simulink model "Project_Sim_Adapt"  (R2025a)
settings: Solver=VariableStepAuto  StartTime=0.0  StopTime=simulation_time  RelTol=1e-3
undefined symbols (not defined in the file): N, omegaB0, pWB0, qWB0, Ts, vWB0, x0, Xref
libraries: robotcorelib x1, uavutilslib x1
settings Model: Creator=franc  LastModifiedBy=franc
settings DebuggingCC: UnderspecifiedInitializationDetection=Classic  MergeDetectMultiDrivingBlocksExec=none
settings ModelReferenceCC: PropagateSignalLabelsOutOfModel=off
settings RTWCC: GPUComputeCapability=3.5

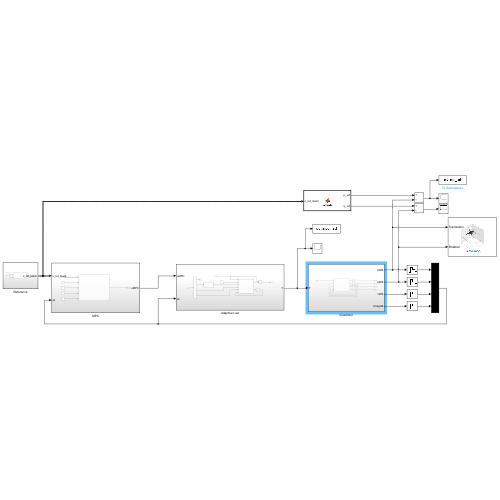
[thumbnail: Simulink's stored preview of the top-level diagram]
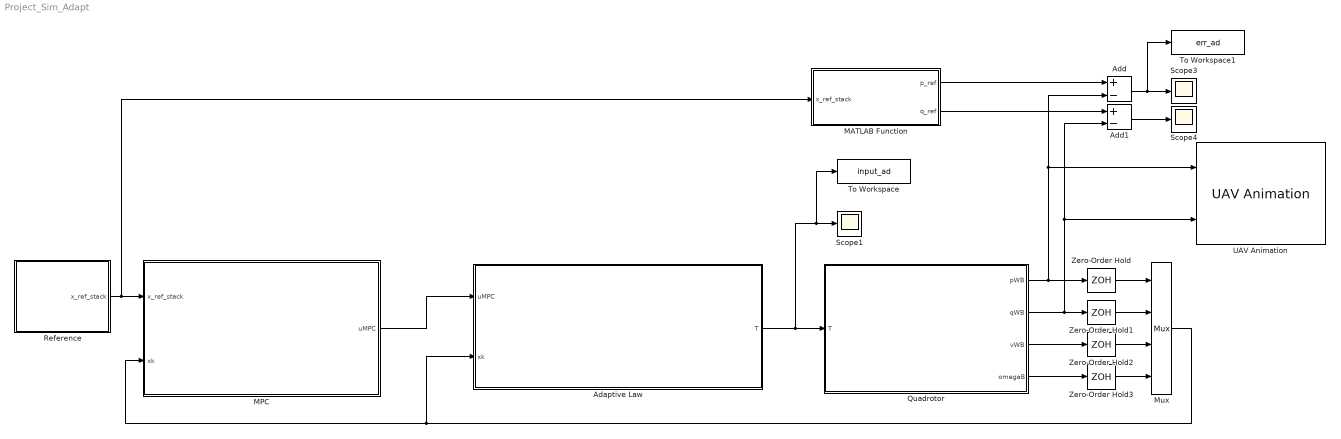
== system Project_Sim_Adapt ==
  Adaptive Law : Subsystem
  Add : Sum  Inputs=+-
  Add1 : Sum  Inputs=+-
  MATLAB Function : MATLAB Function  TreatAsAtomicUnit=on
  MPC : Subsystem
  Mux : Mux
  Quadrotor : Subsystem
  Reference : Subsystem
  Scope1 : Scope
      settings: ActiveDisplayYMinimum=1.7052326467122152  ActiveDisplayYMaximum=1.8134132267959873
  Scope3 : Scope
      settings: ActiveDisplayYMinimum=-0.065328340754687408  ActiveDisplayYMaximum=0.039807612944060038  DataLoggingVariableName=ScopeData4
  Scope4 : Scope
      settings: ActiveDisplayYMinimum=-0.128474772332549  ActiveDisplayYMaximum=0.10839492409722418  DataLoggingVariableName=ScopeData5
  To Workspace : ToWorkspace  VariableName=input_ad  SaveFormat=Structure With Time  SampleTime=-1
  To Workspace1 : ToWorkspace  VariableName=err_ad  SaveFormat=Structure With Time  SampleTime=-1
  UAV Animation : uavutilslib/UAV Animation  NumUAV=1  DynamicUAVConfig=off  UAVType=Multirotor  UAVSize=1  UAVColor=[1 0 0]  UAVTrajectoryAlpha=1  InertialZDirection=Up  RotationFormat=Quaternion  DrawMarkers=off  SampleTime=-1
  Zero-Order Hold{,1..3} (4 alike) : ZeroOrderHold  SampleTime=Ts
  wires:
  Quadrotor/1(pWB) -> UAV Animation/1, Add/2, Zero-Order Hold/1
  Quadrotor/2(qWB) -> UAV Animation/2, Add1/2, Zero-Order Hold1/1
  Quadrotor/3(vWB) -> Zero-Order Hold2/1
  Quadrotor/4(omegaB) -> Zero-Order Hold3/1
  Zero-Order Hold3/1 -> Mux/4
  Zero-Order Hold2/1 -> Mux/3
  Zero-Order Hold1/1 -> Mux/2
  Zero-Order Hold/1 -> Mux/1
  Mux/1 -> Adaptive Law/2(xk), MPC/2(xk)
  Reference/1(x_ref_stack) -> MATLAB Function/1(x_ref_stack), MPC/1(x_ref_stack)
  MATLAB Function/1(p_ref) -> Add/1
  Add/1 -> To Workspace1/1, Scope3/1
  MATLAB Function/2(q_ref) -> Add1/1
  Add1/1 -> Scope4/1
  Adaptive Law/1(T) -> To Workspace/1, Scope1/1, Quadrotor/1(T)
  MPC/1(uMPC) -> Adaptive Law/1(uMPC)

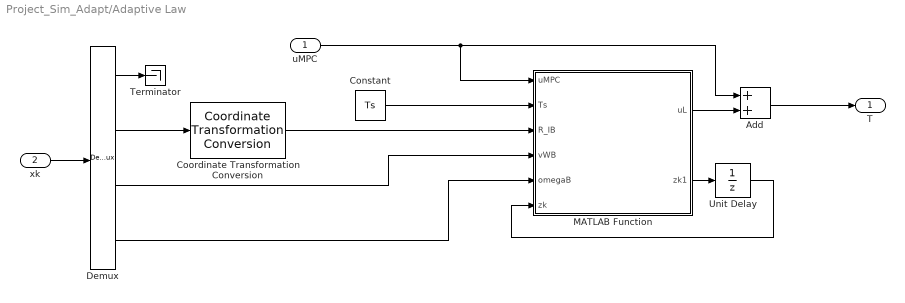
== system Project_Sim_Adapt/Adaptive Law ==
  uMPC : Inport
  xk : Inport  Port=2
  Add : Sum
  Constant : Constant  Value=Ts
  Coordinate Transformation Conversion : robotcorelib/Coordinate Transformation Conversion  InputRepresentation=Quaternion  InputEulerSequence=ZYX  ShowTrVecInputPort=on  OutputRepresentation=Rotation Matrix  OutputEulerSequence=ZYX  ShowTrVecOutputPort=on  SimulateUsing=Interpreted execution
      settings: LibrarySourceBlock=uavutilslib/Coordinate Transformation Conversion
  Demux : Demux  Outputs=[3 4 3 3]
  MATLAB Function : MATLAB Function  TreatAsAtomicUnit=on
  Terminator : Terminator
  Unit Delay : UnitDelay  SampleTime=-1  HasFrameUpgradeWarning=on
  T : Outport
  wires:
  xk/1 -> Demux/1
  Demux/3 -> MATLAB Function/4(vWB)
  Demux/4 -> MATLAB Function/5(omegaB)
  uMPC/1 -> Add/1, MATLAB Function/1(uMPC)
  Demux/1 -> Terminator/1
  Constant/1 -> MATLAB Function/2(Ts)
  Coordinate Transformation Conversion/1 -> MATLAB Function/3(R_IB)
  MATLAB Function/2(zk1) -> Unit Delay/1
  Unit Delay/1 -> MATLAB Function/6(zk)
  Demux/2 -> Coordinate Transformation Conversion/1
  MATLAB Function/1(uL) -> Add/2
  Add/1 -> T/1

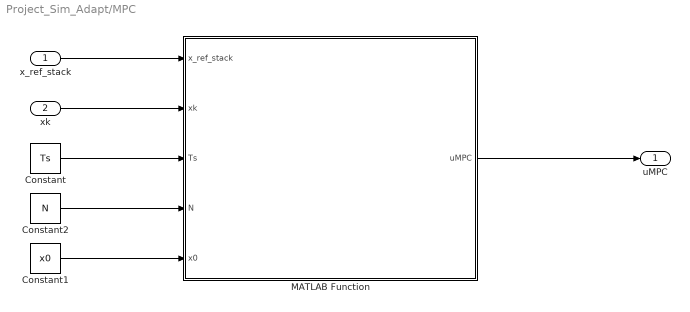
== system Project_Sim_Adapt/MPC ==
  x_ref_stack : Inport
  xk : Inport  Port=2
  Constant : Constant  Value=Ts
  Constant1 : Constant  Value=x0
  Constant2 : Constant  Value=N
  MATLAB Function : MATLAB Function  TreatAsAtomicUnit=on
  uMPC : Outport
  wires:
  Constant/1 -> MATLAB Function/3(Ts)
  Constant1/1 -> MATLAB Function/5(x0)
  xk/1 -> MATLAB Function/2(xk)
  MATLAB Function/1(uMPC) -> uMPC/1
  Constant2/1 -> MATLAB Function/4(N)
  x_ref_stack/1 -> MATLAB Function/1(x_ref_stack)

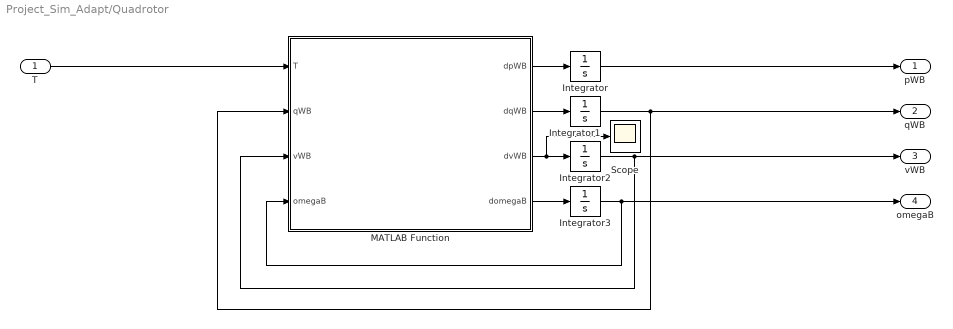
== system Project_Sim_Adapt/Quadrotor ==
  T : Inport
  Integrator : Integrator  InitialCondition=pWB0
  Integrator1 : Integrator  InitialCondition=qWB0
  Integrator2 : Integrator  InitialCondition=vWB0
  Integrator3 : Integrator  InitialCondition=omegaB0
  MATLAB Function : MATLAB Function  TreatAsAtomicUnit=on
  Scope : Scope
      settings: ActiveDisplayYMinimum=-10.516652542372883  ActiveDisplayYMaximum=1.7458474576271188  DataLoggingVariableName=ScopeData2
  pWB : Outport
  qWB : Outport  Port=2
  vWB : Outport  Port=3
  omegaB : Outport  Port=4
  wires:
  T/1 -> MATLAB Function/1(T)
  MATLAB Function/1(dpWB) -> Integrator/1
  MATLAB Function/2(dqWB) -> Integrator1/1
  MATLAB Function/3(dvWB) -> Scope/1, Integrator2/1
  MATLAB Function/4(domegaB) -> Integrator3/1
  Integrator1/1 -> MATLAB Function/2(qWB), qWB/1
  Integrator2/1 -> MATLAB Function/3(vWB), vWB/1
  Integrator3/1 -> MATLAB Function/4(omegaB), omegaB/1
  Integrator/1 -> pWB/1

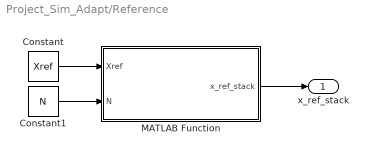
== system Project_Sim_Adapt/Reference ==
  Constant : Constant  Value=Xref
  Constant1 : Constant  Value=N
  MATLAB Function : MATLAB Function  TreatAsAtomicUnit=on  SystemSampleTime=Ts
  x_ref_stack : Outport
  wires:
  Constant1/1 -> MATLAB Function/2(N)
  Constant/1 -> MATLAB Function/1(Xref)
  MATLAB Function/1(x_ref_stack) -> x_ref_stack/1

== matlab function Project_Sim_Adapt/MPC/MATLAB Function ==
  data: x_ref_stack input; xk input size=13; uMPC output size=4; Ts input size=1; N input; x0 input size=13
function uMPC = MPC(x_ref_stack,xk,Ts,N,x0)

% Initialization
persistent ubar x0_guess u0_guess;

u_hover = 0.716*9.81/4; 
if isempty(ubar)
    ubar = u_hover*ones(4,1);
end

% Dimensions
nx = 13;
nu = 4;

% Cost parameters
R = 10*eye(nu);
Q = diag(400*[10 10 200 1 1 1 1 1 1 1 1 1 1]);

% Inequality constraints per time step (input) (H_u*u <= k_u)
rpm_max = 10880;
omega_max = rpm_max*2*pi/60;
u_max = 1.6e-2*omega_max^2;

H_u = [ eye(nu);
      -eye(nu)];
k_u = [ u_max*ones(nu,1);
       zeros(nu,1)];

% Inequality constraints per time step (state, fictional) (H_x*x <= k_x)
x_min = -1e6*ones(nx,1);
x_max = 1e6*ones(nx,1);
H_x = [ eye(nx);
       -eye(nx)];
k_x = [ x_max;
       -x_min ];

% System dynamics (Computation of the linearized system around the current state)
[Ak,Bk,ck] = lin_fdyn_central(xk, ubar, Ts);

% Inequality constraints for the whole horizon (A*z <= b)
% z = [x0,x1,...,xN-1,xN,u0,u1,...,uN-1]'
Ax = kron(eye(N+1), H_x);
bx = repmat(k_x, N+1, 1);
Au = kron(eye(N), H_u);
bu = repmat(k_u, N, 1);

A = blkdiag(Ax,Au);
b = [bx;bu];

% Equality constraints
Aeq=zeros(nx*(N+1),nx*(N+1)+nu*N);
beq=zeros(nx*(N+1),1);

for k=0:N-1 % Linearized system dynamics constraints 
    Aeq(nx*k+1:nx*(k+1),1:nx*(N+1))=[zeros(nx,nx*k),Ak,-eye(nx),zeros(nx,nx*(N-1-k))];
    Aeq(nx*k+1:nx*(k+1),nx*(N+1)+1:end)=[zeros(nx,nu*k),Bk,zeros(nx,nu*(N-1-k))];
    beq(nx*k+1:nx*(k+1)) = -ck;
end

% Initial condition constraints
Aeq(nx*N+1:nx*(N+1),:)=[eye(nx),zeros(nx,nu*N+nx*N)];
beq(nx*N+1:nx*(N+1))=xk;

% Cost function
Qstack = kron(eye(N+1), Q); % Q, but for the whole horizon
Rstack = kron(eye(N), R); % R, but for the whole horizon
    
HQP = blkdiag(Qstack,Rstack); % Overall cost

u_ref_stack = repmat(u_hover*ones(nu,1), N, 1); % Constant reference on the input
fQP = -HQP * [x_ref_stack; u_ref_stack]; % x and u centered on their references

% solver parameters
if isempty(x0_guess)
    x0_guess = repmat(x0,N+1,1);
end
if isempty(u0_guess)
    u0_guess = repmat(u_hover*ones(nu,1),N,1);
end
tol_opt       = 1e-8;
options = optimoptions('quadprog', ...
                       'Algorithm', 'active-set', ...
                       'MaxIterations', 10000, ...
                       'OptimalityTolerance', tol_opt, ...
                       'StepTolerance', tol_opt);

% optimization
solutionOL = quadprog(HQP,fQP,A,b,Aeq,beq,[],[],[x0_guess;u0_guess],options);

% Derive the optimal predicted state and input sequence
x_OL_tilde = solutionOL(1:nx*(N+1),1);
u_OL_tilde = solutionOL(nx*(N+1)+1:end,1);
x_OL = reshape(x_OL_tilde,nx,N+1);
u_OL = reshape(u_OL_tilde,nu,N);

% Prepare warmstart solution for next time step 
x0_guess = [x_OL_tilde(nx+1:end);zeros(nx,1)];
u0_guess = [u_OL_tilde(nu+1:end);zeros(nu,1)];

% Imposing MPC action
uMPC = u_OL(:,1);
ubar = uMPC;

%% functions for system dynamics

    function [Ak,Bk,ck] = lin_fdyn_central(xbar, ubar, dt) % system dynamics linearization

        % Retrieving the Nonlinear system dynamics
        nnx = numel(xbar);
        nnu = numel(ubar);
        f0 = fRK4(xbar, ubar, dt);

        % denominator settings
        hx = (eps^(1/3))*max(1, abs(xbar));
        hu = (eps^(1/3))*max(1, abs(ubar));

        % Matrices initialization
        Ak = zeros(nnx);
        Bk = zeros(nnx,nnu);

        for i = 1:nnx % Ak computation
            dx = zeros(nnx,1);
            dx(i) = hx(i);
            fp = fRK4(xbar+dx, ubar, dt);
            fm = fRK4(xbar-dx, ubar, dt);
            Ak(:,i) = (fp-fm)/(2*hx(i));
        end

        for j = 1:nnu % Bk computation
            du = zeros(nnu,1);
            du(j) = hu(j);
            fp = fRK4(xbar, ubar+du, dt);
            fm = fRK4(xbar, ubar-du, dt);
            Bk(:,j) = (fp-fm)/(2*hu(j));
       end

       ck = f0-Ak*xbar-Bk*ubar; % Residual computation
    end


    function xk1 = fRK4(xk,uk,deltaT) % Runge-Kutta 4th order discretization
        k1 = f(xk,uk);
        k2 = f(xk+deltaT/2*k1,uk);
        k3 = f(xk+deltaT/2*k2,uk);
        k4 = f(xk+deltaT*k3,uk);
        xk1 = xk+deltaT/6*(k1+2*k2+2*k3+k4);
    end

    function dotx = f(x,u) % Nonlinear Nominal system dynamics (see Plant code for details)
    g = 9.81;
    g_vec = [0 0 -g]';

    T0 = u(1);
    T1 = u(2);
    T2 = u(3);
    T3 = u(4);

    TB = [0 0 T0+T1+T2+T3]';
    m = 0.716;
    
    Jx = 0.007;
    Jy = Jx;
    Jz = 0.012;

    J = diag([Jx,Jy,Jz]);

    xx = zeros(4,1);
    yy = zeros(4,1);
    dxx = zeros(4,1);
    dyy = zeros(4,1);

    l = 0.17;
    theta = [0 pi/2 pi -pi/2]';
    for i=1:4
       xx(i)=l*cos(theta(i));
       yy(i)=l*sin(theta(i));
    end
    for i=1:4
        dxx(i)=abs(yy(i));
        dyy(i)=abs(xx(i));
    end
    cT = 1.6e-2;
    P = [-dxx(1) -dxx(2) dxx(3) dxx(4);
         dyy(1) -dyy(2) -dyy(3) dyy(4)
         -cT     cT    -cT    cT];

    tauB = P*[T0 T1 T2 T3]';

    pWB = x(1:3);
    qWB = x(4:7);
    vWB = x(8:10);
    omegaB = x(11:13);

    dpWB = vWB;
    dqWB = quatmultiply(qWB,[0 omegaB'/2]');
    dvWB = quaternion_product(qWB,TB/m)+g_vec;
    domegaB = inv(J)*(tauB - cross(omegaB, J*omegaB));

    dotx = [dpWB;dqWB;dvWB;domegaB];


        function res = quaternion_product(q, vec) % quaternion * vector
        q = q/ norm(q);
        q_conj = [q(1) -q(2) -q(3) -q(4)]';
        q_vec = [0 vec']';
        res = quatmultiply(q, q_vec);
        res = quatmultiply(res,q_conj);
        res = res(2:4);
    end


    function q_out = quatmultiply(q1, q2) % quaternion multiplication

    qw1 = q1(1); qx1 = q1(2); qy1 = q1(3); qz1 = q1(4);
    qw2 = q2(1); qx2 = q2(2); qy2 = q2(3); qz2 = q2(4);

    q_out = [qw1*qw2 - qx1*qx2 - qy1*qy2 - qz1*qz2; 
             qw1*qx2 + qx1*qw2 + qy1*qz2 - qz1*qy2; 
             qw1*qy2 - qx1*qz2 + qy1*qw2 + qz1*qx2; 
             qw1*qz2 + qx1*qy2 - qy1*qx2 + qz1*qw2];
    end
    end
end

== matlab function Project_Sim_Adapt/Quadrotor/MATLAB Function ==
  data: T input size=4; qWB input size=4; vWB input size=3; dpWB output size=3; dqWB output size=4; dvWB output size=3; domegaB output size=3; omegaB input size=3
function [dpWB,dqWB,dvWB,domegaB] = dynamics(T,qWB,vWB,omegaB)

    % gravity term
    g = 9.81;
    g_vec = [0 0 -g]';

    % thrusts
    T0 = T(1);
    T1 = T(2);
    T2 = T(3);
    T3 = T(4);
    TB = [0 0 T0+T1+T2+T3]';
    
    % mass
    m = 0.716;
    
    % Inertia
    Jx = 0.007;
    Jy = Jx;
    Jz = 0.012;
    J = diag([Jx,Jy,Jz]);

    % Allocation Matrix computation
    l = 0.17;
    theta = [0 pi/2 pi -pi/2]';
    xx = zeros(4,1);
    yy = zeros(4,1);
    dxx = zeros(4,1);
    dyy = zeros(4,1);
    for i=1:4
       xx(i)=l*cos(theta(i));
       yy(i)=l*sin(theta(i));
    end
    for i=1:4
        dxx(i)=abs(yy(i));
        dyy(i)=abs(xx(i));
    end
    cT = 1.6e-2;
    P = [-dxx(1) -dxx(2) dxx(3) dxx(4);
         dyy(1) -dyy(2) -dyy(3) dyy(4)
         -cT     cT    -cT    cT];

    tauB = P*[T0 T1 T2 T3]';

    % disturbed values
    m = m+0.660;
    J = 2*J;
    lr = 0.17;
    lf = 0.17*0.75;
    for i=1:2
       xx(i)=lr*cos(theta(i));
       yy(i)=lr*sin(theta(i));
    end
    for i=3:4
       xx(i)=lf*cos(theta(i));
       yy(i)=lf*sin(theta(i));
    end
    for i=1:4
        dxx(i)=abs(yy(i));
        dyy(i)=abs(xx(i));
    end
    P = [-dxx(1) -dxx(2) dxx(3) dxx(4);
         dyy(1) -dyy(2) -dyy(3) dyy(4)
         -cT     cT    -cT    cT];
    tauB = P*[T0 T1 T2 T3]';

    % model dynamics
    dpWB = vWB;
    dqWB = quatmultiply(qWB,[0 omegaB'/2]');
    dvWB = quaternion_product(qWB,TB/m)+g_vec;
    domegaB = inv(J)*(tauB - cross(omegaB, J*omegaB));


    function res = quaternion_product(q, vec) % quaternion * vector
        q = q/ norm(q);
        q_conj = [q(1) -q(2) -q(3) -q(4)]';
        q_vec = [0 vec']';
        tmp_1 = quatmultiply(q, q_vec);
        tmp_2 = quatmultiply(tmp_1,q_conj);
        res = tmp_2(2:4);
    end


    function q_out = quatmultiply(q1, q2) % quaternion product

    qw1 = q1(1); qx1 = q1(2); qy1 = q1(3); qz1 = q1(4);
    qw2 = q2(1); qx2 = q2(2); qy2 = q2(3); qz2 = q2(4);

    q_out = [qw1*qw2 - qx1*qx2 - qy1*qy2 - qz1*qz2;
             qw1*qx2 + qx1*qw2 + qy1*qz2 - qz1*qy2; 
             qw1*qy2 - qx1*qz2 + qy1*qw2 + qz1*qx2; 
             qw1*qz2 + qx1*qy2 - qy1*qx2 + qz1*qw2];
    end

end

== matlab function Project_Sim_Adapt/Reference/MATLAB Function ==
  data: Xref input; x_ref_stack output size=[13*(N+1), 1]; N input
function x_ref_stack = buildRefStack(Xref, N)

% This code simply retrieves the whole trajectory and gives as output the
% trajectory between current time and the end of the horizon for the MPC

    persistent k;
    if isempty(k)
        k = 1;
    end

    nx = 13;
    Ttot = size(Xref, 2);
    k_end = k + N;
    if k_end > Ttot
        k_end = Ttot;
    end

    Xslice = Xref(:, k:k_end);
    missing = (N+1) - size(Xslice,2);
    if missing > 0
        lastcol = Xslice(:, end);
        Xslice = [Xslice, repmat(lastcol, 1, missing)];
    end
    x_ref_stack = reshape(Xslice, nx*(N+1), 1);

    if k < Ttot
        k = k + 1;
    end
end

== matlab function Project_Sim_Adapt/MATLAB Function ==
  data: x_ref_stack input; p_ref output; q_ref output
function [p_ref,q_ref] = getRefs(x_ref_stack)
    p_ref = x_ref_stack(1:3);
    q_ref = x_ref_stack(4:7);
end

== matlab function Project_Sim_Adapt/Adaptive Law/MATLAB Function ==
  data: uMPC input size=4; Ts input size=1; R_IB input size=[3 3]; uL output size=4; vWB input size=3; omegaB input size=3; zk input size=6; zk1 output size=6
function [uL,zk1] = Adaption(uMPC, Ts, R_IB, vWB, omegaB, zk)

persistent u_old;
if isempty(u_old)
    u_old = zeros(4,1);
end

% list of nominal model parameters
g_grav = [0 0 -9.81]';
m = 0.716;
Jx = 0.007;
Jy = Jx;
Jz = 0.012;
J = diag([Jx,Jy,Jz]);
xx = zeros(4,1);
yy = zeros(4,1);
dxx = zeros(4,1);
dyy = zeros(4,1);
l = 0.17;
theta = [0 pi/2 pi -pi/2]';
for i=1:4
   xx(i)=l*cos(theta(i));
   yy(i)=l*sin(theta(i));
end
for i=1:4
    dxx(i)=abs(yy(i));
    dyy(i)=abs(xx(i));
end
cT = 1.6e-2;
P = [-dxx(1) -dxx(2) dxx(3) dxx(4);
     dyy(1) -dyy(2) -dyy(3) dyy(4)
      -cT      cT     -cT      cT];
T0 = uMPC(1);
T1 = uMPC(2);
T2 = uMPC(3);
T3 = uMPC(4);
tauB = P*[T0 T1 T2 T3]';
TB = T0+T1+T2+T3;

% Computation of Cd (Matrix of linear drag coefficients)
width  = 0.02;
height = 0.02;
Sx = 2*l*height;
Sy = 2*l*height;
Sz = 4*l*width;
rho = 1.225;
CD  = 1.0;
v0 = 1.0;
Cx = rho*Sx*CD*v0;
Cy = rho*Sy*CD*v0;
Cz = rho*Sz*CD*v0;
Cd = diag([Cx, Cy, Cz]);

% cutoff frequency
omega_co = 15;

% Rotation vectors from the body frame
ex_B = R_IB(:,1);
ey_B = R_IB(:,2);
ez_B = R_IB(:,3);

% Reduced state variable
z = [vWB; omegaB];
z_tilde = zk-z;

% Matrix of adaption gains
As = diag(5*2.56*[1 1 1 1 1 1]);

% Definition of PHI
PHI = As\(expm(As*Ts)-eye(size(As))); 

% Definition of mi
mi = expm(As*Ts)*z_tilde;

% Uncertainty of matched and unmatched components
g = [ez_B/m ez_B/m ez_B/m ez_B/m; J\P];
g_ort = [ex_B/m ey_B/m; zeros(3,1) zeros(3,1)];
G = [g g_ort];

% Matched and unmatched uncertainties computation
sigma_hat = -eye(6)*G\(PHI\mi);
sigma_hat_m = sigma_hat(1:4);
sigma_hat_um = sigma_hat(5:6);

% Setting uL as result of a first order digital filter
uL = u_old*exp(-omega_co*Ts)-sigma_hat_m*(1-exp(-omega_co*Ts));

% Adaptive dynamics function
f = [g_grav+TB/m*ez_B-Cd*vWB; J\tauB-cross(omegaB,J*omegaB)];

% Discrete dynamics of zk
zk1 = zk+(f+g*(uL+sigma_hat_m)+g_ort*sigma_hat_um+As*z_tilde)*Ts;
